simulink model "upsample"  (R2024a)
settings: Solver=VariableStepAuto  StartTime=0.0  StopTime=10.0  RelTol=1e-3
libraries: dsphdlsigops2 x2, dspsnks4 x1, dspvision x1
settings Model: Creator=fermata  LastModifiedBy=fermata

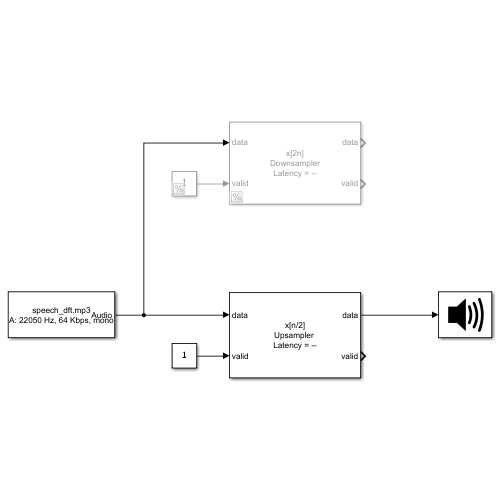
[thumbnail: Simulink's stored preview of the top-level diagram]
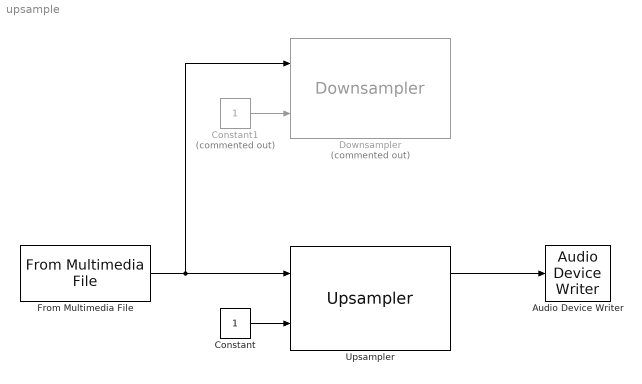
== system upsample ==
  Audio Device Writer : dspsnks4/Audio Device Writer  Driver=ALSA  Device=Default  InheritSampleRate=on  SampleRate=44100  BitDepth=16-bit integer  BufferSize=4096  NumBuffers=10  DefaultOutputChannelMapping=on  OutputChannelMapping=1:2  OutputNumUnderrunSamples=off  DriverIdx=8  DeviceWarnFlag=''
  Constant : Constant  OutDataTypeStr=boolean
  Constant1 : Constant  Commented=on  OutDataTypeStr=boolean
  Downsampler : dsphdlsigops2/Downsampler  Commented=on  DownsampleFactor=2  SampleOffset=0  SimulateUsing=Code generation  ResetInputPort=off
  From Multimedia File : dspvision/From Multimedia File  inputFilename=speech_dft.mp3  readRange=[1 Inf]  loop=on  numPlays=inf  outputStreams=Audio only  videoDataType=single  audioDataType=double  inheritSampleTime=on  userDefinedSampleTime=1/30  noAudioOutput=off  isIntensityVideo=off  fourcc=RGB  colorVideoFormat=Separate color signals  outputEOF=off  dataOrg=Column-major  audioFrameSize=1  computeAudioFrameSize=off  outSamplingMode=Sample based
      settings: LibrarySourceBlock=audiosources/From Multimedia File
  Upsampler : dsphdlsigops2/Upsampler  UpsampleFactor=2  SampleOffset=0  NumCycles=1  SimulateUsing=Code generation  ResetInputPort=off  ReadyPort=off
  wires:
  From Multimedia File/1 -> Downsampler/1, Upsampler/1
  Upsampler/1 -> Audio Device Writer/1
  Constant/1 -> Upsampler/2
  Constant1/1 -> Downsampler/2
